simulink model "P1_Sim_Simulink3"  (R2022a)
settings: Solver=FixedStepAuto  StartTime=0.0  StopTime=tf  FixedStep=dt  RelTol=1e-3
values from neighbouring files (symbols this model uses):
  Model = 2    [syms_math.m]
  x_initial = [0.5 ; 0 ; deg2rad(30) ; 0]    [syms_math.m]
  xd = [0.5 , 0 , 0 , 0]    [syms_math.m]
settings Model: Creator=brendoncallen  LastModifiedBy=anw0060
settings SolverCC: AlgebraicLoopSolver=TrustRegion
settings DataIOCC: ReturnWorkspaceOutputs=off
settings DebuggingCC: UnconnectedInputMsg=warning  UnconnectedOutputMsg=warning  UnconnectedLineMsg=warning  SFMachineParentedDataDiag=warning  ArithmeticOperatorsInVariantConditions=warning
settings SFSimCC: SimUseLocalCustomCode=off  CustomCodeUndefinedFunction=UseInterfaceOnly
settings RTWCC: RTWUseLocalCustomCode=off  DLArmComputeVersion=19.05

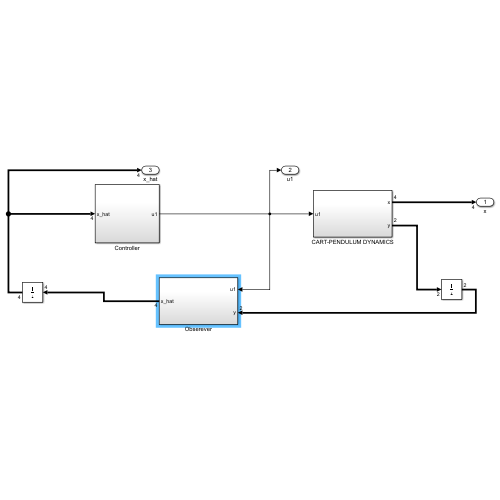
[thumbnail: Simulink's stored preview of the top-level diagram]
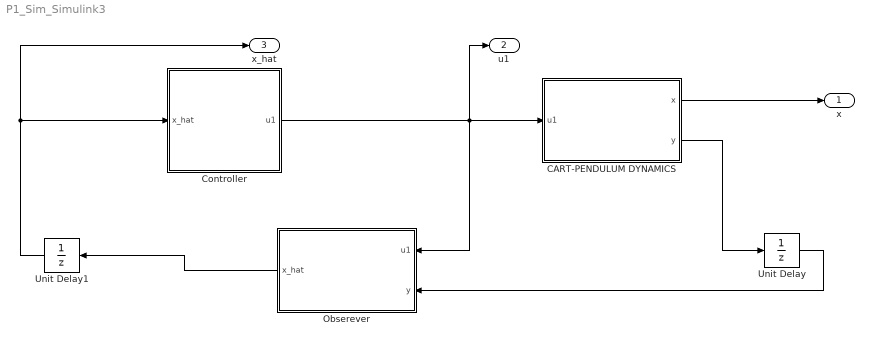
== system P1_Sim_Simulink3 ==
  CART-PENDULUM DYNAMICS : Subsystem
  Controller : Subsystem
  Obserever : Subsystem
  Unit Delay : UnitDelay  SampleTime=-1  HasFrameUpgradeWarning=on
  Unit Delay1 : UnitDelay  SampleTime=-1  HasFrameUpgradeWarning=on
  x : Outport  VectorParamsAs1DForOutWhenUnconnected=off
  u1 : Outport  Port=2  VectorParamsAs1DForOutWhenUnconnected=off
  x_hat : Outport  Port=3
  wires:
  CART-PENDULUM DYNAMICS/1(x) -> x/1
  Controller/1(u1) -> u1/1, Obserever/1(u1), CART-PENDULUM DYNAMICS/1(u1)
  CART-PENDULUM DYNAMICS/2(y) -> Unit Delay/1
  Unit Delay/1 -> Obserever/2(y)
  Obserever/1(x_hat) -> Unit Delay1/1
  Unit Delay1/1 -> x_hat/1, Controller/1(x_hat)

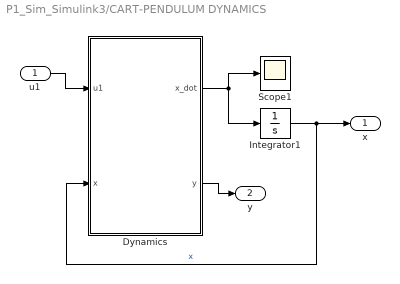
== system P1_Sim_Simulink3/CART-PENDULUM DYNAMICS ==
  u1 : Inport
  Dynamics : MATLAB Function  TreatAsAtomicUnit=on
  Integrator1 : Integrator  InitialCondition=x_initial
  Scope1 : Scope
  x : Outport  VectorParamsAs1DForOutWhenUnconnected=off
  y : Outport  Port=2
  wires:
  Dynamics/1(x_dot) -> Scope1/1, Integrator1/1
  Integrator1/1 -> x/1, Dynamics/2(x)  "x"
  u1/1 -> Dynamics/1(u1)
  Dynamics/2(y) -> y/1

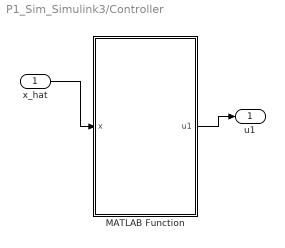
== system P1_Sim_Simulink3/Controller ==
  x_hat : Inport
  MATLAB Function : MATLAB Function  TreatAsAtomicUnit=on
  u1 : Outport  VectorParamsAs1DForOutWhenUnconnected=off
  wires:
  x_hat/1 -> MATLAB Function/1(x)
  MATLAB Function/1(u1) -> u1/1

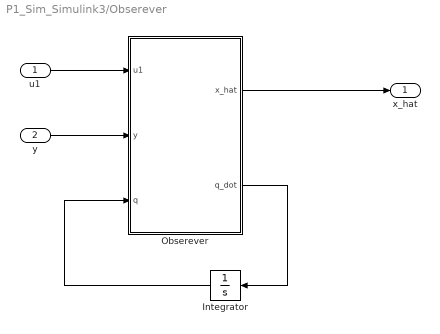
== system P1_Sim_Simulink3/Obserever ==
  u1 : Inport
  y : Inport  Port=2
  Integrator : Integrator
  Obserever : MATLAB Function  TreatAsAtomicUnit=on
  x_hat : Outport  VectorParamsAs1DForOutWhenUnconnected=off
  wires:
  u1/1 -> Obserever/1(u1)
  y/1 -> Obserever/2(y)
  Obserever/1(x_hat) -> x_hat/1
  Obserever/2(q_dot) -> Integrator/1
  Integrator/1 -> Obserever/3(q)

== matlab function P1_Sim_Simulink3/Obserever/Obserever ==
  data: u1 input size=1; x_hat output size=4; y input; L2 parameter; q input; q_dot output
function [x_hat,q_dot]  = dynamics(u1,y,L2,q)

% Inverted Pendulum-Cart System

%   x is the state vector of [x; x_dot; phi; phi_dot],  4x1 vector
%   u is the control input the the cart,                1x1 scalar
%   phi is measured from the upward vertical in the CCW direction.
%   u is the control input in the positive right direction
%   x is measured relative to a desired x-cooridnate

%% System Parameters
M = 0.5;     %Mass of the Cart [kg]
m = 0.2;     %Mass of the pendulum [kg]
b = 0.1;     %Coeff of friction for the cart
l = 0.3;     %Length to pendulum CoM
I = 0.006;   %Moment of inertia of the pendulum
g = 9.8;  %Gravitational Const. [m/s^2]

ml = m*l; % To reduce # of calculations

%% System Model
   
    a1=M*l^2*m+I*M+I*m;
    A = [0 , 1 , 0 , 0; ... 
        0 , (-I*b-b*l^2*m)/a1 , (m^2*g*l^2)/a1 , 0; ...
        0 , 0 , 0 , 1; ...
        0 , (-b*l*m)/a1 , (M*g*l*m+m^2*g*l)/a1 , 0];
    B = [0 ; (I+l^2*m)/a1 ; 0 ; (l*m)/a1];
    C=[1 , 0 , 0 , 0; 0 , 0 , 1 , 0];
    D=[0 ; 0];
 
   T=[C; 0 , 1 , 0 , 0 ;0  , 0 , 0, 1 ];
   A_t=T*A*inv(T);
   A1=A_t(1:2,1:2);
   A2=A_t(1:2,3:4);
   A3=A_t(3:4,1:2);
   A4=A_t(3:4,3:4);

   B_t=T*B;
   B1=B_t(1:2,1);
   B2=B_t(3:4,1);

   q_dot=(A3-L2*A1)*y+(A4-L2*A2)*(q+L2*y)+(B2-L2*B1)*u1;
   z_hat=q+L2*y;

   x_hat=inv(T)*[y;z_hat];


end

== matlab function P1_Sim_Simulink3/Controller/MATLAB Function ==
  data: x input size=4; u1 output size=1; K parameter
function u1 = controller(x, K)

    u1 = -K*x;

end

== matlab function P1_Sim_Simulink3/CART-PENDULUM DYNAMICS/Dynamics ==
  data: u1 input size=1; x input size=4; x_dot output size=4; Model parameter size=1; xd parameter; y output
function [x_dot, y] = dynamics(u1,x,Model, xd)

% Inverted Pendulum-Cart System

%   x is the state vector of [x; x_dot; phi; phi_dot],  4x1 vector
%   u is the control input the the cart,                1x1 scalar
%   phi is measured from the upward vertical in the CCW direction.
%   u is the control input in the positive right direction
%   x is measured relative to a desired x-cooridnate

%% System Parameters
M = 0.5;     %Mass of the Cart [kg]
m = 0.2;     %Mass of the pendulum [kg]
b = 0.1;     %Coeff of friction for the cart
l = 0.3;     %Length to pendulum CoM
I = 0.006;   %Moment of inertia of the pendulum
g = 9.8;  %Gravitational Const. [m/s^2]

ml = m*l; % To reduce # of calculations

%% System Model

x1 = x(1);
x2 = x(2);
x3 = x(3);
x4 = x(4);

if Model == 1 %Linear Model
   
    a1=M*l^2*m+I*M+I*m;
    A = [0 , 1 , 0 , 0; ... 
        0 , (-I*b-b*l^2*m)/a1 , (m^2*g*l^2)/a1 , 0; ...
        0 , 0 , 0 , 1; ...
        0 , (-b*l*m)/a1 , (M*g*l*m+m^2*g*l)/a1 , 0];
    B = [0 ; (I+l^2*m)/a1 ; 0 ; (l*m)/a1];

    x_dot = A*x + B*u1;
else % Nonlinear Model


    x_dot_1 = x2;
    x_dot_2 = -((I*b*x2-u1*I-u1*(l^2)*m+b*(l^2)*m*x2+(l^3)*(m^2)*(x4^2)*sin(x3)-g*(l^2)*(m^2)*cos(x3)*sin(x3)+I*l*m*(x4^2)*sin(x3))/(-(l^2)*(m^2)*(cos(x3)^2)+(l^2)*(m^2)+M*(l^2)*m+I*m+I*m));
    x_dot_3 = x4;
    x_dot_4 = (l*m*(-l*m*cos(x3)*sin(x3)*(x4^2)+u1*cos(x3)+M*g*sin(x3)-b*x2*cos(x3)+g*m*sin(x3)))/(-(l^2)*(m^2)*(cos(x3)^2)+(l^2)*(m^2)+M*(l^2)*m+I*m+I*m);

    x_dot = [x_dot_1;x_dot_2;x_dot_3;x_dot_4];

    
end
C=[1 , 0 , 0 , 0; 0 , 0 , 1 , 0];
D=[0 ; 0];
y=C*x+D*u1;
end
